simulink model "Exp4_MODEL_Trolley"  (R2023b)
settings: Solver=ode3  StartTime=0.0  StopTime=Time(end)  FixedStep=0.001  RelTol=1e-3
undefined symbols (not defined in the file): A, c_D, g, k_M, k_St, k_Te, m_trans_St, m_trans_Te, mu_R_St, mu_R_Te, r_DG, rho_A, v_rot, x_rot
settings Model: Creator=tunkarlu  LastModifiedBy=tunkarlu

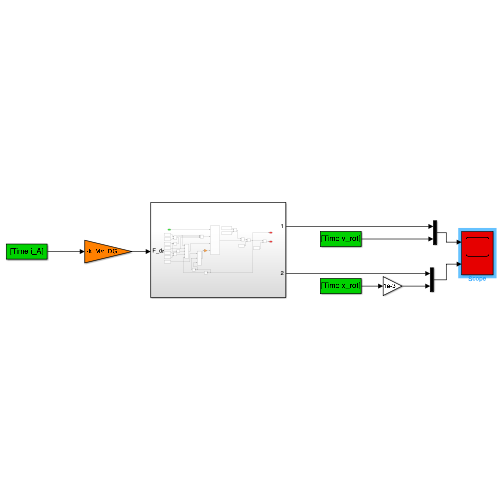
[thumbnail: Simulink's stored preview of the top-level diagram]
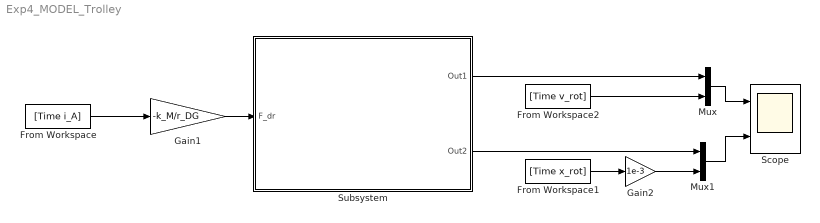
== system Exp4_MODEL_Trolley ==
  From Workspace : FromWorkspace  VariableName=[Time i_A]
  From Workspace1 : FromWorkspace  VariableName=[Time x_rot]
  From Workspace2 : FromWorkspace  VariableName=[Time v_rot]
  Gain1 : Gain  Gain=-k_M/r_DG
  Gain2 : Gain  Gain=1e-3
  Mux : Mux  Inputs=2
  Mux1 : Mux  Inputs=2
  Scope : Scope  NumInputPorts=2
  Subsystem : Subsystem
  wires:
  From Workspace/1 -> Gain1/1
  From Workspace2/1 -> Mux/2
  From Workspace1/1 -> Gain2/1
  Gain2/1 -> Mux1/2
  Mux/1 -> Scope/1
  Subsystem/1(Out1) -> Mux/1
  Gain1/1 -> Subsystem/1(F_dr)
  Subsystem/2(Out2) -> Mux1/1
  Mux1/1 -> Scope/2

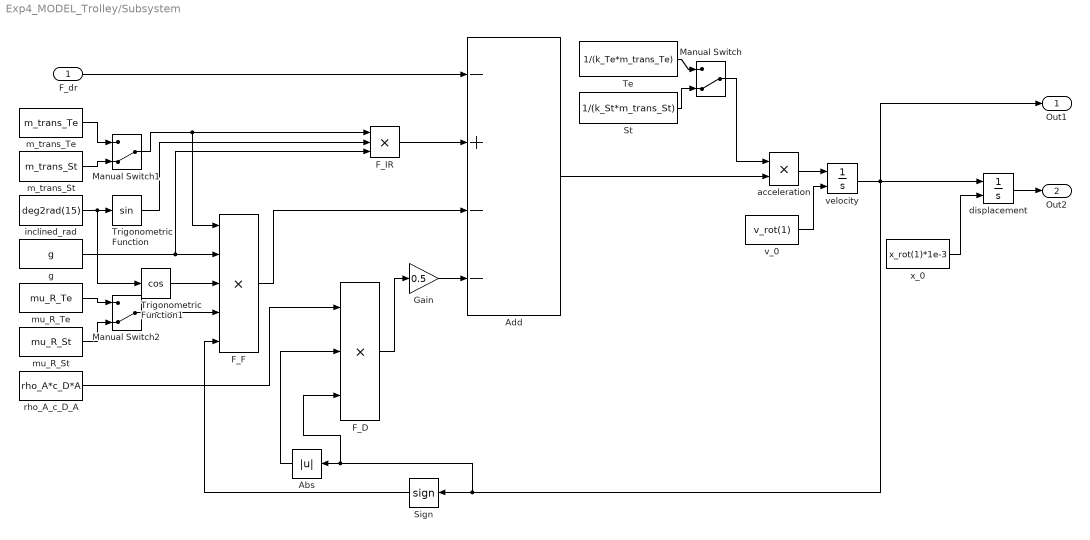
== system Exp4_MODEL_Trolley/Subsystem ==
  F_dr : Inport
  Abs : Abs  SaturateOnIntegerOverflow=off
  Add : Sum  Inputs=-+--
  F_D : Product  Inputs=3
  F_F : Product  Inputs=5
  F_IR : Product  Inputs=3
  Gain : Gain  Gain=0.5
  Manual Switch : ManualSwitch  CurrentSetting=0
  Manual Switch1 : ManualSwitch  CurrentSetting=0
  Manual Switch2 : ManualSwitch  CurrentSetting=0
  Sign : Signum
  St : Constant  Value=1/(k_St*m_trans_St)
  Te : Constant  Value=1/(k_Te*m_trans_Te)
  Trigonometric Function : Trigonometry
  Trigonometric Function1 : Trigonometry  Operator=cos
  acceleration : Product
  displacement : Integrator  InitialConditionSource=external
  g : Constant  Value=g
  inclined_rad : Constant  Value=deg2rad(15)
  m_trans_St : Constant  Value=m_trans_St
  m_trans_Te : Constant  Value=m_trans_Te
  mu_R_St : Constant  Value=mu_R_St
  mu_R_Te : Constant  Value=mu_R_Te
  rho_A_c_D_A : Constant  Value=rho_A*c_D*A
  v_0 : Constant  Value=v_rot(1)
  velocity : Integrator  InitialConditionSource=external
  x_0 : Constant  Value=x_rot(1)*1e-3
  Out1 : Outport
  Out2 : Outport  Port=2
  wires:
  Te/1 -> Manual Switch/1
  St/1 -> Manual Switch/2
  acceleration/1 -> velocity/1
  Manual Switch/1 -> acceleration/1
  Add/1 -> acceleration/2
  F_dr/1 -> Add/1
  m_trans_Te/1 -> Manual Switch1/1
  m_trans_St/1 -> Manual Switch1/2
  inclined_rad/1 -> Trigonometric Function1/1, Trigonometric Function/1
  Manual Switch1/1 -> F_F/1, F_IR/1
  Trigonometric Function/1 -> F_IR/2
  g/1 -> F_F/2, F_IR/3
  mu_R_Te/1 -> Manual Switch2/1
  mu_R_St/1 -> Manual Switch2/2
  Manual Switch2/1 -> F_F/4
  Trigonometric Function1/1 -> F_F/3
  velocity/1 -> displacement/1, F_D/3, Abs/1, Sign/1, Out1/1
  Sign/1 -> F_F/5
  F_F/1 -> Add/3
  Gain/1 -> Add/4
  F_D/1 -> Gain/1
  rho_A_c_D_A/1 -> F_D/1
  displacement/1 -> Out2/1
  x_0/1 -> displacement/2
  v_0/1 -> velocity/2
  Abs/1 -> F_D/2
  F_IR/1 -> Add/2
